simulink model "_old_SRManL4_ZADANIE1_MODEL"  (R2018a)
settings: Solver=ode45  StartTime=0.0  StopTime=tend  MaxStep=Tp  RelTol=1e-3
undefined symbols (not defined in the file): D, eta, initConditionsPos, initConditionsVel, invR, Km, Lambda, omega1, omega2, Qd01, Qd02, Qd1, Qd11, Qd12, Qd1const, Qd2, Qd21, Qd22, Qd2const, Qd31, Qd32
libraries: simulink x2
settings Model: Creator=szymon  LastModifiedBy=szymon

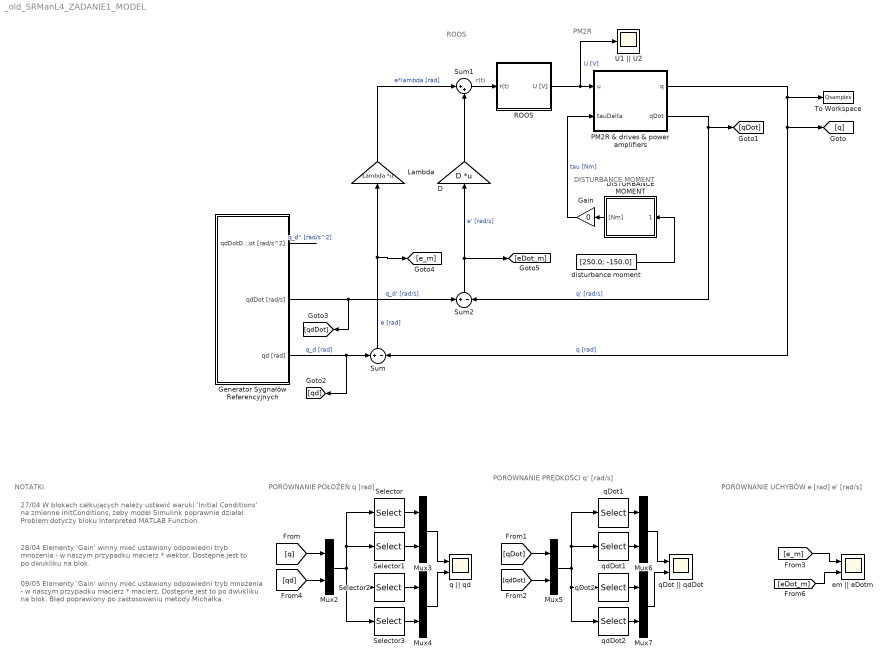
== system _old_SRManL4_ZADANIE1_MODEL ==
  note: PM2R
  note: ROOS
  note: DISTURBANCE MOMENT
  note: PORÓWNANIE POŁOŻEŃ
      | q [rad]
  note: NOTATKI
  note: 27/04 W blokach całkujących należy ustawić waruki
      | 'Initial Conditions' na zmienne initConditions, żeby model
      | Simulink poprawnie działał. Problem dotyczy bloku
      | Interpreted MATLAB Function.
  note: 28/04 Elementy 'Gain' winny mieć ustawiony odpowiedni tryb
      | mnożenia - w naszym przypadku macierz * wektor.
      | Dostępne jest to po dwukliku na blok.
  note: PORÓWNANIE PRĘDKOŚCI
      | q' [rad/s]
  note: 09/05 Elementy 'Gain' winny mieć ustawiony odpowiedni tryb
      | mnożenia - w naszym przypadku macierz * macierz.
      | Dostępne jest to po dwukliku na blok. Błąd poprawiony po
      | zastosowaniu metody Michałka.
  note: PORÓWNANIE UCHYBÓW
      | e  [rad]
      | e' [rad/s]
  D : Gain  Gain=D  Multiplication=Matrix(K*u) (u vector)
  DISTURBANCE MOMENT : Subsystem
  Gain : Gain  Gain=0
  Generator Sygnałów Referencyjnych : Subsystem
  Lambda : Gain  Gain=Lambda  Multiplication=Matrix(K*u) (u vector)
  Mux{2..7} (6 alike) : Mux  Inputs=2
  PM2R & drives & power amplifiers : Subsystem
  ROOS : Subsystem
  Selector : Selector  InputPortWidth=4  IndexOptions=Index vector (dialog)  Indices=[1]  OutputSizes=1
  Selector1 : Selector  InputPortWidth=4  IndexOptions=Index vector (dialog)  Indices=[3]  OutputSizes=1
  Selector2 : Selector  InputPortWidth=4  IndexOptions=Index vector (dialog)  Indices=[2]  OutputSizes=1
  Selector3 : Selector  InputPortWidth=4  IndexOptions=Index vector (dialog)  Indices=[4]  OutputSizes=1
  Sum : Sum  Inputs=+-
  Sum1 : Sum  Inputs=|++
  Sum2 : Sum  Inputs=+-
  To Workspace : ToWorkspace  VariableName=Qsamples  SampleTime=-1
  U1 || U2 : Scope
  disturbance moment : Constant  Value=[250.0; -150.0]
  em || eDotm : Scope  NumInputPorts=2
  q || qd : Scope  NumInputPorts=2
  qDot || qdDot : Scope  NumInputPorts=2
  qDot1 : Selector  InputPortWidth=4  IndexOptions=Index vector (dialog)  Indices=[1]  OutputSizes=1
  qDot2 : Selector  InputPortWidth=4  IndexOptions=Index vector (dialog)  Indices=[2]  OutputSizes=1
  qdDot1 : Selector  InputPortWidth=4  IndexOptions=Index vector (dialog)  Indices=[3]  OutputSizes=1
  qdDot2 : Selector  InputPortWidth=4  IndexOptions=Index vector (dialog)  Indices=[4]  OutputSizes=1
  wires:
  PM2R & drives & power amplifiers/2(qDot) -> [qDot], Sum2/2  "q' [rad/s]"
  PM2R & drives & power amplifiers/1(q) -> To Workspace/1, [q], Sum/2  "q [rad]"
  [q] -> Mux2/1
  [qd] -> Mux2/2
  Selector/1 -> Mux3/1
  Selector1/1 -> Mux3/2
  Selector2/1 -> Mux4/1
  Selector3/1 -> Mux4/2
  Mux2/1 -> Selector3/1, Selector2/1, Selector1/1, Selector/1
  Mux3/1 -> q || qd/1
  Mux4/1 -> q || qd/2
  qDot2/1 -> Mux7/1
  Mux6/1 -> qDot || qdDot/1
  Mux7/1 -> qDot || qdDot/2
  qdDot2/1 -> Mux7/2
  [qDot] -> Mux5/1
  qdDot1/1 -> Mux6/2
  [qdDot] -> Mux5/2
  qDot1/1 -> Mux6/1
  Mux5/1 -> qdDot2/1, qDot2/1, qdDot1/1, qDot1/1
  Generator Sygnałów Referencyjnych/2(qdDot [rad/s]) -> Sum2/1, [qdDot]  "q_d' [rad/s]"
  Sum2/1 -> D/1, [eDot_m]  "e' [rad/s]"
  Sum/1 -> [e_m], Lambda/1  "e [rad]"
  [e_m] -> em || eDotm/1
  Generator Sygnałów Referencyjnych/3(qd [rad]) -> Sum/1, [qd]  "q_d [rad]"
  [eDot_m] -> em || eDotm/2
  Gain/1 -> PM2R & drives & power amplifiers/2(tauDelta)  "tau [Nm]"
  Lambda/1 -> Sum1/1  "e*lambda [rad]"
  Generator Sygnałów Referencyjnych/1(qdDotDot [rad/s^2]) -> ?  "q_d'' [rad/s^2]"
  disturbance moment/1 -> DISTURBANCE MOMENT/1(in [Nm])
  DISTURBANCE MOMENT/1("[Nm]") -> Gain/1
  ROOS/1(U [V]) -> PM2R & drives & power amplifiers/1(u), U1 || U2/1  "U [V]"
  Sum1/1 -> ROOS/1(r(t))  "r(t)"
  D/1 -> Sum1/2

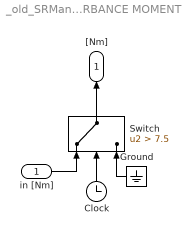
== system _old_SRManL4_ZADANIE1_MODEL/DISTURBANCE MOMENT ==
  in [Nm] : Inport
  Clock : Clock
  Ground : Ground
  Switch : Switch  Criteria=u2 > Threshold  Threshold=7.5
  "[Nm]" : Outport
  wires:
  Clock/1 -> Switch/2
  Ground/1 -> Switch/3
  in [Nm]/1 -> Switch/1
  Switch/1 -> "[Nm]"/1

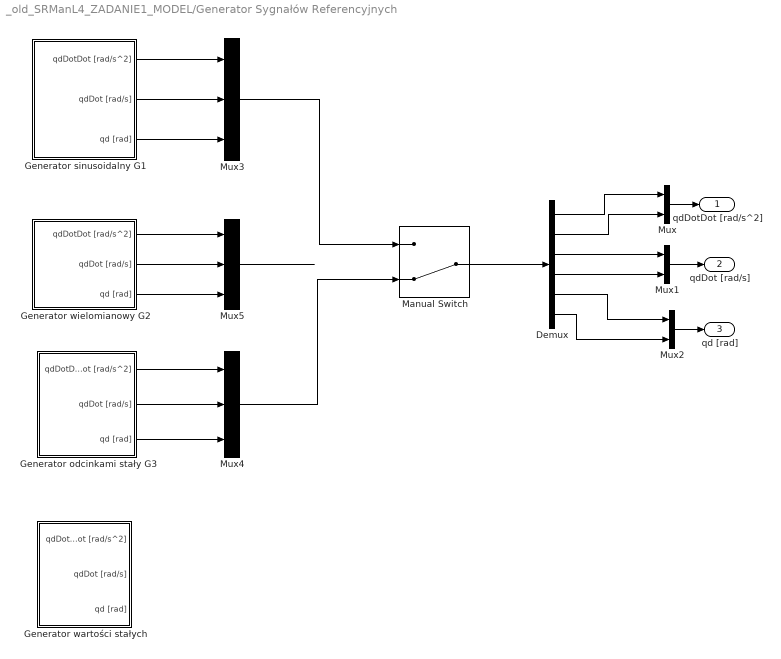
== system _old_SRManL4_ZADANIE1_MODEL/Generator Sygnałów Referencyjnych ==
  Demux : Demux  Outputs=6
  "Generator odcinkami stały G3 " : Subsystem
  Generator sinusoidalny G1 : Subsystem
  Generator wielomianowy G2 : Subsystem
  Generator wartości stałych : Subsystem
  Manual Switch : ManualSwitch  CurrentSetting=0
  Mux : Mux  Inputs=2
  Mux1 : Mux  Inputs=2
  Mux2 : Mux  Inputs=2
  Mux3 : Mux  Inputs=3
  Mux4 : Mux  Inputs=3
  Mux5 : Mux  Inputs=3
  qdDotDot [rad/s^2] : Outport
  qdDot [rad/s] : Outport  Port=2
  qd [rad] : Outport  Port=3
  wires:
  Mux/1 -> qdDotDot [rad/s^2]/1
  Mux2/1 -> qd [rad]/1
  Mux1/1 -> qdDot [rad/s]/1
  Manual Switch/1 -> Demux/1
  Demux/1 -> Mux/1
  Demux/2 -> Mux/2
  Demux/3 -> Mux1/1
  Demux/4 -> Mux1/2
  Demux/5 -> Mux2/1
  Demux/6 -> Mux2/2
  Generator sinusoidalny G1/2(qdDot [rad/s]) -> Mux3/2
  Generator sinusoidalny G1/1(qdDotDot [rad/s^2]) -> Mux3/1
  Generator sinusoidalny G1/3(qd [rad]) -> Mux3/3
  Mux3/1 -> Manual Switch/1
  "Generator odcinkami stały G3 "/1(qdDotDot [rad/s^2]) -> Mux4/1
  "Generator odcinkami stały G3 "/2(qdDot [rad/s]) -> Mux4/2
  "Generator odcinkami stały G3 "/3(qd [rad]) -> Mux4/3
  Mux4/1 -> Manual Switch/2
  Generator wielomianowy G2/1(qdDotDot [rad/s^2]) -> Mux5/1
  Generator wielomianowy G2/2(qdDot [rad/s]) -> Mux5/2
  Generator wielomianowy G2/3(qd [rad]) -> Mux5/3
  Mux5/1 -> ?

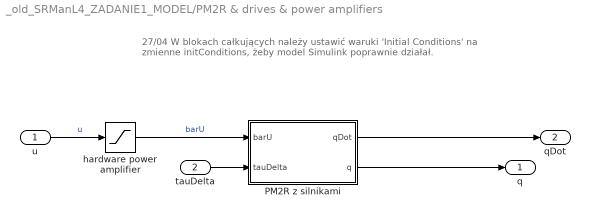
== system _old_SRManL4_ZADANIE1_MODEL/PM2R & drives & power amplifiers ==
  note: 27/04 W blokach całkujących należy ustawić waruki 'Initial Conditions' na
      | zmienne initConditions, żeby model Simulink poprawnie działał.
  u : Inport
  tauDelta : Inport  Port=2
  PM2R z silnikami : Subsystem
  hardware power amplifier : Saturate  UpperLimit=24.0  LowerLimit=-24.0
  q : Outport
  qDot : Outport  Port=2
  wires:
  u/1 -> hardware power amplifier/1  "u"
  PM2R z silnikami/1(qDot) -> qDot/1
  PM2R z silnikami/2(q) -> q/1
  tauDelta/1 -> PM2R z silnikami/2(tauDelta)
  hardware power amplifier/1 -> PM2R z silnikami/1(barU)  "barU"

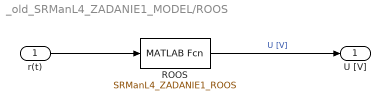
== system _old_SRManL4_ZADANIE1_MODEL/ROOS ==
  r(t) : Inport
  ROOS : MATLABFcn  MATLABFcn=SRManL4_ZADANIE1_ROOS
  U [V] : Outport
  wires:
  ROOS/1 -> U [V]/1  "U [V]"
  r(t)/1 -> ROOS/1

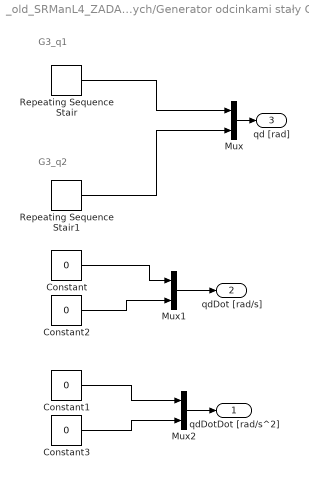
== system _old_SRManL4_ZADANIE1_MODEL/Generator Sygnałów Referencyjnych/Generator odcinkami stały G3  ==
  note: G3_q2
  note: G3_q1
  Constant{,1..3} (4 alike) : Constant  Value=0
  Mux : Mux  Inputs=2
  Mux1 : Mux  Inputs=2
  Mux2 : Mux  Inputs=2
  Repeating Sequence Stair : simulink/Sources/Repeating Sequence Stair  OutValues=[Qd1const 0].'  tsamp=Ta  OutMin=[]  OutMax=[]  OutDataTypeStr=double  OutputDataTypeScalingMode=double  OutDataType=fixdt(0,8)  ConRadixGroup=Best Precision: Vector-wise  OutScaling=2^-12
  Repeating Sequence Stair1 : simulink/Sources/Repeating Sequence Stair  OutValues=[Qd2const 0].'  tsamp=Tb  OutMin=[]  OutMax=[]  OutDataTypeStr=double  OutputDataTypeScalingMode=double  OutDataType=fixdt(0,8)  ConRadixGroup=Best Precision: Vector-wise  OutScaling=2^-12
  qdDotDot [rad/s^2] : Outport
  qdDot [rad/s] : Outport  Port=2
  qd [rad] : Outport  Port=3
  wires:
  Constant/1 -> Mux1/1
  Repeating Sequence Stair1/1 -> Mux/2
  Repeating Sequence Stair/1 -> Mux/1
  Mux/1 -> qd [rad]/1
  Constant1/1 -> Mux2/1
  Constant2/1 -> Mux1/2
  Constant3/1 -> Mux2/2
  Mux2/1 -> qdDotDot [rad/s^2]/1
  Mux1/1 -> qdDot [rad/s]/1

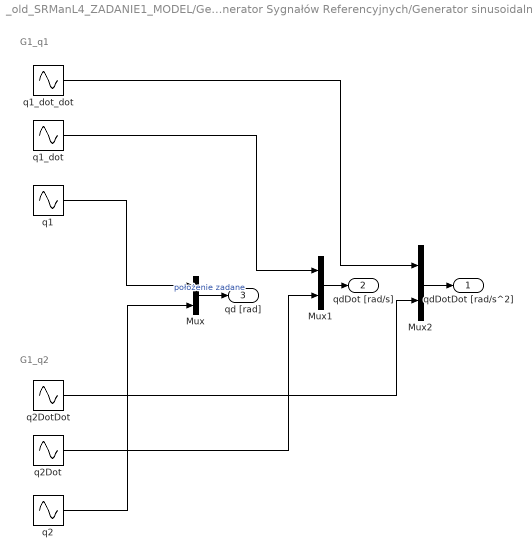
== system _old_SRManL4_ZADANIE1_MODEL/Generator Sygnałów Referencyjnych/Generator sinusoidalny G1 ==
  note: G1_q1
  note: G1_q2
  Mux : Mux  Inputs=2
  Mux1 : Mux  Inputs=2
  Mux2 : Mux  Inputs=2
  "q1 " : Sin  Amplitude=Qd1  Frequency=omega1  SampleTime=0
  q1_dot : Sin  Amplitude=omega1*Qd1  Frequency=omega1  Phase=pi/2  SampleTime=0
  "q1_dot_dot " : Sin  Amplitude=-omega1^2*Qd1  Frequency=omega1  SampleTime=0
  q2 : Sin  Amplitude=Qd2  Frequency=omega2  SampleTime=0
  q2Dot : Sin  Amplitude=omega2*Qd2  Frequency=omega2  Phase=pi/2  SampleTime=0
  "q2DotDot " : Sin  Amplitude=-omega2^2*Qd2  Frequency=omega2  SampleTime=0
  qdDotDot [rad/s^2] : Outport
  qdDot [rad/s] : Outport  Port=2
  qd [rad] : Outport  Port=3
  wires:
  Mux1/1 -> qdDot [rad/s]/1
  Mux2/1 -> qdDotDot [rad/s^2]/1
  "q1_dot_dot "/1 -> Mux2/1
  "q2DotDot "/1 -> Mux2/2
  q2Dot/1 -> Mux1/2
  q1_dot/1 -> Mux1/1
  q2/1 -> Mux/2
  "q1 "/1 -> Mux/1
  Mux/1 -> qd [rad]/1  "położenie zadane"

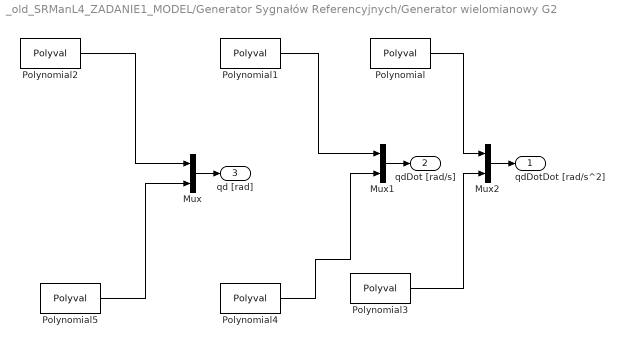
== system _old_SRManL4_ZADANIE1_MODEL/Generator Sygnałów Referencyjnych/Generator wielomianowy G2 ==
  Mux : Mux  Inputs=2
  Mux1 : Mux  Inputs=2
  Mux2 : Mux  Inputs=2
  Polynomial : Polyval  Coefs=[6*Qd31*t, 2*Qd21]
  Polynomial1 : Polyval  Coefs=[3*Qd31*t.^2, 2*Qd21*t, Qd11]
  Polynomial2 : Polyval  Coefs=[Qd31*t.^3, Qd21*t.^2, Qd11*t, Qd01]
  Polynomial3 : Polyval  Coefs=[6*Qd32*t, 2*Qd22]
  Polynomial4 : Polyval  Coefs=[3*Qd32*t.^2, 2*Qd22*t, Qd12]
  Polynomial5 : Polyval  Coefs=[Qd32*t.^3, Qd22*t.^2, Qd12*t, Qd02]
  qdDotDot [rad/s^2] : Outport
  qdDot [rad/s] : Outport  Port=2
  qd [rad] : Outport  Port=3
  wires:
  Polynomial/1 -> Mux2/1
  Polynomial1/1 -> Mux1/1
  Polynomial2/1 -> Mux/1
  Polynomial3/1 -> Mux2/2
  Polynomial5/1 -> Mux/2
  Polynomial4/1 -> Mux1/2
  Mux/1 -> qd [rad]/1
  Mux1/1 -> qdDot [rad/s]/1
  Mux2/1 -> qdDotDot [rad/s^2]/1

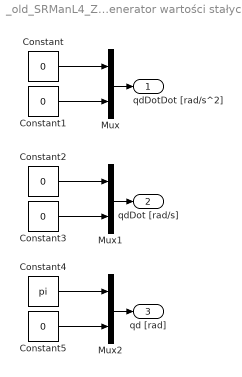
== system _old_SRManL4_ZADANIE1_MODEL/Generator Sygnałów Referencyjnych/Generator wartości stałych ==
  Constant{,1..3,5} (5 alike) : Constant  Value=0
  Constant4 : Constant  Value=pi
  Mux : Mux  Inputs=2
  Mux1 : Mux  Inputs=2
  Mux2 : Mux  Inputs=2
  qdDotDot [rad/s^2] : Outport
  qdDot [rad/s] : Outport  Port=2
  qd [rad] : Outport  Port=3
  wires:
  Constant/1 -> Mux/1
  Mux/1 -> qdDotDot [rad/s^2]/1
  Constant1/1 -> Mux/2
  Constant2/1 -> Mux1/1
  Constant3/1 -> Mux1/2
  Mux1/1 -> qdDot [rad/s]/1
  Constant4/1 -> Mux2/1
  Constant5/1 -> Mux2/2
  Mux2/1 -> qd [rad]/1

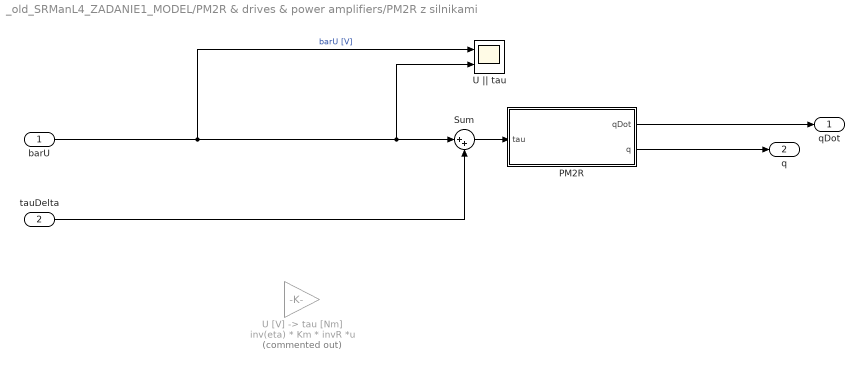
== system _old_SRManL4_ZADANIE1_MODEL/PM2R & drives & power amplifiers/PM2R z silnikami ==
  barU : Inport
  tauDelta : Inport  Port=2
  PM2R : Subsystem
  Sum : Sum  Inputs=|++
  "U [V] -> tau [Nm]" : Gain  Commented=on  Gain=inv(eta) * Km * invR  Multiplication=Matrix(K*u)
  U || tau : Scope  NumInputPorts=2
  qDot : Outport
  q : Outport  Port=2
  wires:
  PM2R/2(q) -> q/1
  PM2R/1(qDot) -> qDot/1
  barU/1 -> U || tau/2, Sum/1, U || tau/1  "barU [V]"
  Sum/1 -> PM2R/1(tau)
  tauDelta/1 -> Sum/2

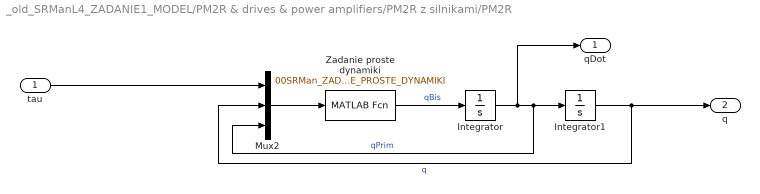
== system _old_SRManL4_ZADANIE1_MODEL/PM2R & drives & power amplifiers/PM2R z silnikami/PM2R ==
  tau : Inport
  Integrator : Integrator  InitialCondition=initConditionsVel
  Integrator1 : Integrator  InitialCondition=initConditionsPos
  Mux2 : Mux  Inputs=3
  Zadanie proste dynamiki : MATLABFcn  MATLABFcn=00SRMan_ZADANIE_PROSTE_DYNAMIKI
  qDot : Outport
  q : Outport  Port=2
  wires:
  Mux2/1 -> Zadanie proste dynamiki/1
  Integrator1/1 -> q/1, Mux2/2  "q"
  Integrator/1 -> qDot/1, Mux2/3, Integrator1/1  "qPrim"
  Zadanie proste dynamiki/1 -> Integrator/1  "qBis"
  tau/1 -> Mux2/1
